simulink model "mainModel"  (R2022b)
settings: Solver=VariableStepAuto  StartTime=0.0  StopTime=10.0  RelTol=1e-3
settings Model: Creator=Mario Bertelli  LastModifiedBy=Mario Bertelli

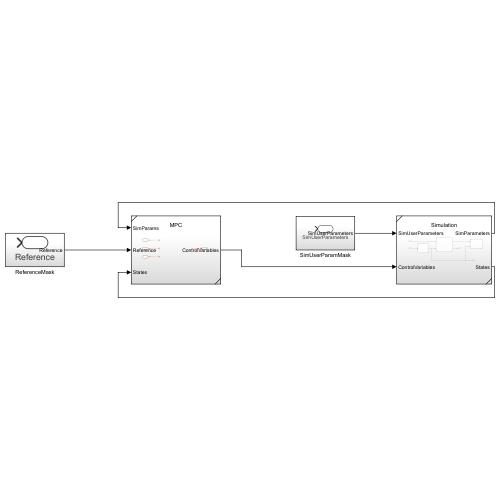
[thumbnail: Simulink's stored preview of the top-level diagram]
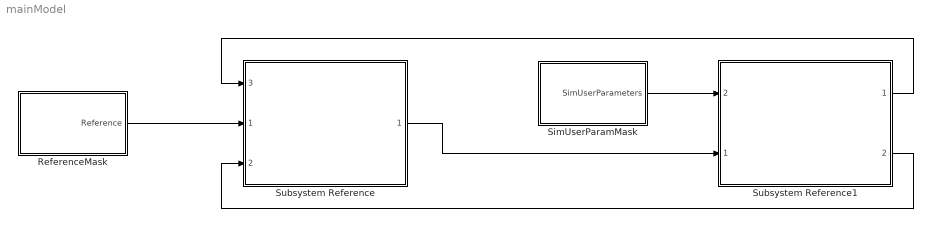
== system mainModel ==
  ReferenceMask : Subsystem
  SimUserParamMask : Subsystem
  Subsystem Reference : Subsystem  ReferencedSubsystem=MPC
      settings: PortSchema="{\"entries\":[{\"content\":{\"sides\":[{\"content\":{\"connectorIds\":[\"In3\",\"In1\",\"In2\"]},\"type\":\"ConnectorPlacement.EquallySpacedRectSide\",\"uuid\":\"b44a1ff6-b0d2-4057-a5af-3b4dc6e07acc\"},{\"content\":{\"connectorIds\":[\"Out1\"],\"side\":\"RIGHT\"},\"type\":\"ConnectorPlacement.EquallySpacedRectSide\",\"uuid\":\"ab0ec655-40b4-4190-ab2a-ad3e59642fb1\"},{\"content\":{\"connectorIds\":[],\"side\":\"TOP\"},\"type\":\"ConnectorPlacement.EquallySpacedRectSide\",\"uuid\":\"cb292ea1-0bc0-4840-9a89-51c5b1b370e0\"}]},\"type\":\"ConnectorPlacement.EquallySpacedConnector\",\"uuid\":\"9b18ca3c-b641-4e4e-b93d-63680c5ca799\"}],\"packageUris\":[\"http://schema.mathworks.com/mf0/Connector/R2020b\"],\"version\":\"1.0\"}"
  Subsystem Reference1 : Subsystem  ReferencedSubsystem=Simulation
      settings: PortSchema="{\"entries\":[{\"content\":{\"sides\":[{\"content\":{\"connectorIds\":[\"In2\",\"In1\"]},\"type\":\"ConnectorPlacement.EquallySpacedRectSide\",\"uuid\":\"01c8b9c1-56d7-4050-b5fb-6d9c8034245e\"},{\"content\":{\"connectorIds\":[\"Out1\",\"Out2\"],\"side\":\"RIGHT\"},\"type\":\"ConnectorPlacement.EquallySpacedRectSide\",\"uuid\":\"18ebbf47-1e2e-49a4-8f33-bdc9f37a46af\"},{\"content\":{\"connectorIds\":[],\"side\":\"TOP\"},\"type\":\"ConnectorPlacement.EquallySpacedRectSide\",\"uuid\":\"dccb08d6-820c-420e-b040-0966249e8e89\"}]},\"type\":\"ConnectorPlacement.EquallySpacedConnector\",\"uuid\":\"3cdccb69-d0b7-44c8-a0a2-462917338e25\"}],\"packageUris\":[\"http://schema.mathworks.com/mf0/Connector/R2020b\"],\"version\":\"1.0\"}"
  wires:
  Subsystem Reference1/2 -> Subsystem Reference/2
  Subsystem Reference/1 -> Subsystem Reference1/1
  Subsystem Reference1/1 -> Subsystem Reference/3
  ReferenceMask/1(Reference) -> Subsystem Reference/1
  SimUserParamMask/1(SimUserParameters) -> Subsystem Reference1/2

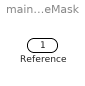
== system mainModel/ReferenceMask ==
  Reference : Outport

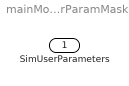
== system mainModel/SimUserParamMask ==
  SimUserParameters : Outport
